simulink model "test"  (R2016a)
settings: Solver=VariableStepAuto  StartTime=0.0  StopTime=10.0  RelTol=1e-3
values from neighbouring files (symbols this model uses):
  A = eye(2)    [main.m]
  B = eye(2)*dt    [main.m]
  D = zeros(6,1)    [GPSGlobal.m]    (also in KalmanGain.m)
  dt = 0.1    [main.m]    (also in master_dcl.m; master_dclZACK.m; try1.m)
  R = 0.5    [main.m]    (also in master_dcl.m = 0.002; master_dclZACK.m = 0.002; try1.m = 0.002)
undefined symbols (not defined in the file or in its folder): C, Discrete, P0, Time
libraries: ctrlSharedLib x2
settings Model: Creator=Giammario  LastModifiedBy=Giammario

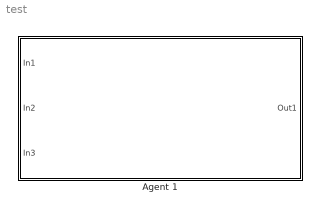
== system test ==
  Agent 1 : Subsystem

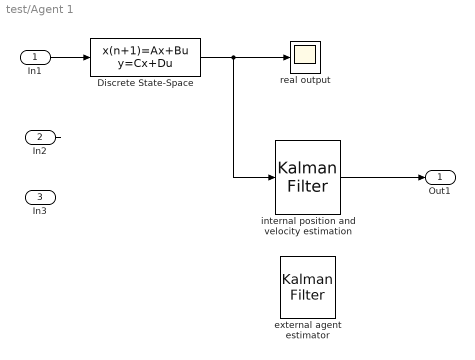
== system test/Agent 1 ==
  In1 : Inport
  In2 : Inport  Port=2
  In3 : Inport  Port=3
  Discrete State-Space : DiscreteStateSpace  A=A  B=B  C=C  D=D  X0=P0(:,1)  SampleTime=dt
  external agent estimator : ctrlSharedLib/Kalman Filter  TimeDomain=Discrete-Time  UseCurrentEstimator=on  ModelSource=LTI State-Space Variable  ModelSourceVariable=ss(0.95,1,1,0,1)  A=0.95  B=1  C=1  D=0  NumberOfStates=1  NumberOfInputs=1  NumberOfOutputs=1  InitialEstimateSource=Dialog  X0=0  P0=10  UseK=off  UseGH=off  NumberOfProcessNoiseInputs=1  G=1  TimeInvariantG=on  H=0  TimeInvariantH=on  Q=0.05  TimeInvariantQ=on  R=1  TimeInvariantR=on  N=0  TimeInvariantN=on  AddInputPort=on  AddEnablePort=off  OutputEstimatedY=off  OutputP=off  Ts=-1
  internal position and velocity estimation : ctrlSharedLib/Kalman Filter  TimeDomain=Discrete-Time  UseCurrentEstimator=on  ModelSource=Individual A, B, C, D matrices  ModelSourceVariable=ss(0.95,1,1,0,1)  A=A  B=B  C=C  D=0  NumberOfStates=4  NumberOfInputs=2  NumberOfOutputs=4  InitialEstimateSource=Dialog  X0=[20,20,10,10]  P0=10  UseK=off  UseGH=off  NumberOfProcessNoiseInputs=1  G=1  TimeInvariantG=on  H=0  TimeInvariantH=on  Q=Q  TimeInvariantQ=on  R=R  TimeInvariantR=on  N=0  TimeInvariantN=on  AddInputPort=off  AddEnablePort=off  OutputEstimatedY=off  OutputP=off  Ts=-1
  real output : Scope
  Out1 : Outport
  wires:
  Discrete State-Space/1 -> real output/1, internal position and velocity estimation/1
  internal position and velocity estimation/1 -> Out1/1
  In1/1 -> Discrete State-Space/1
  In2/1 -> ?
